simulink model "Doubling_Logic"  (R2021b)
settings: Solver=VariableStepAuto  StartTime=0.0  StopTime=10.0  RelTol=1e-3
settings Model: Creator=HP  LastModifiedBy=HP

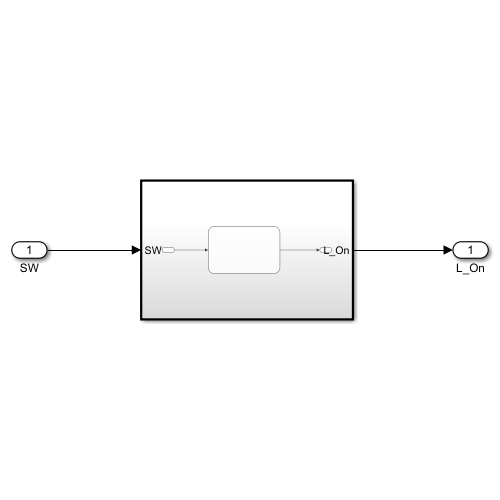
[thumbnail: Simulink's stored preview of the top-level diagram]
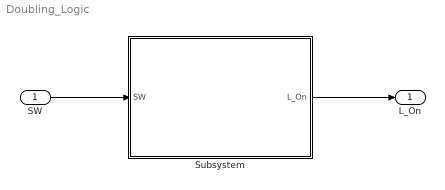
== system Doubling_Logic ==
  SW : Inport
  Subsystem : Subsystem  TreatAsAtomicUnit=on
  L_On : Outport
  wires:
  SW/1 -> Subsystem/1(SW)
  Subsystem/1(L_On) -> L_On/1

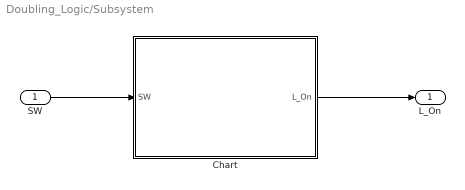
== system Doubling_Logic/Subsystem ==
  SW : Inport
  Chart : Stateflow chart  TreatAsAtomicUnit=on
  L_On : Outport
  wires:
  Chart/1(L_On) -> L_On/1
  SW/1 -> Chart/1(SW)

== stateflow chart Doubling_Logic/Subsystem/Chart ==
  state Off
    en: L_On = 0;
    state Fault
    state Normal
    Fault -> Normal
    (default) -> Normal
  state Doubling
    state Off
    state On
    Doubling.On -> Doubling.Off [order 2] : [SW<0]
    Doubling.Off -> Doubling.On [order 2] : [SW>0]
  state On
    en:
    L_On = 1;
  (default) -> Off
  Doubling -> Fault : after(0.3, sec)
  Doubling.Off -> Off [order 1] : after(0.1, sec)
  Off -> Doubling.On : [SW>0]
  On -> Doubling.Off : [SW<0]
  Doubling.On -> On [order 1] : after(0.1, sec)
  data: L_On output; SW input
